simulink subsystem "SubSystemVereinzelung"  (R2020b)
settings: Solver=VariableStepAuto  StartTime=0.0  StopTime=10.0  RelTol=1e-3
libraries: simulink x6, eeGeneralControl x5
settings Model: Creator=kaebi  LastModifiedBy=kaebi

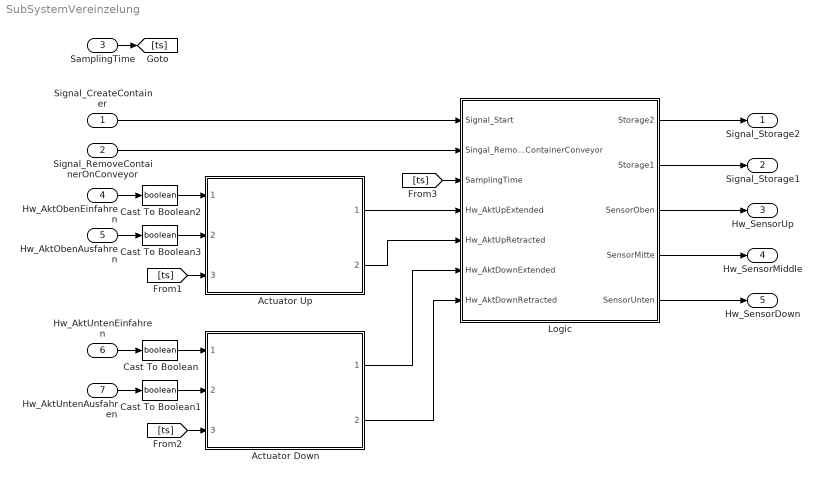
== system SubSystemVereinzelung ==
  Signal_CreateContainer : Inport
  Signal_RemoveContainerOnConveyor : Inport  Port=2
  SamplingTime : Inport  Port=3
  Hw_AktObenEinfahren : Inport  Port=4
  Hw_AktObenAusfahren : Inport  Port=5
  Hw_AktUntenEinfahren : Inport  Port=6
  Hw_AktUntenAusfahren : Inport  Port=7
  Actuator Down : Subsystem  ReferencedSubsystem=SubSystemHubmagnetVereinzelung
  Actuator Up : Subsystem  ReferencedSubsystem=SubSystemHubmagnetVereinzelung
  Cast To Boolean{,1..3} (4 alike) : DataTypeConversion  OutDataTypeStr=boolean
  Logic : Subsystem
  Signal_Storage2 : Outport
  Signal_Storage1 : Outport  Port=2
  Hw_SensorUp : Outport  Port=3
  Hw_SensorMiddle : Outport  Port=4
  Hw_SensorDown : Outport  Port=5
  wires:
  [ts] -> Actuator Up/3
  [ts] -> Actuator Down/3
  SamplingTime/1 -> [ts]
  Logic/5(SensorUnten) -> Hw_SensorDown/1
  Logic/4(SensorMitte) -> Hw_SensorMiddle/1
  Logic/3(SensorOben) -> Hw_SensorUp/1
  Logic/2(Storage1) -> Signal_Storage1/1
  Logic/1(Storage2) -> Signal_Storage2/1
  Signal_CreateContainer/1 -> Logic/1(Signal_Start)
  [ts] -> Logic/3(SamplingTime)
  Signal_RemoveContainerOnConveyor/1 -> Logic/2(Singal_RemoveContainerConveyor)
  Actuator Up/1 -> Logic/4(Hw_AktUpExtended)
  Actuator Up/2 -> Logic/5(Hw_AktUpRetracted)
  Actuator Down/1 -> Logic/6(Hw_AktDownExtended)
  Actuator Down/2 -> Logic/7(Hw_AktDownRetracted)
  Hw_AktObenEinfahren/1 -> Cast To Boolean2/1
  Hw_AktObenAusfahren/1 -> Cast To Boolean3/1
  Cast To Boolean2/1 -> Actuator Up/1
  Cast To Boolean3/1 -> Actuator Up/2
  Hw_AktUntenEinfahren/1 -> Cast To Boolean/1
  Hw_AktUntenAusfahren/1 -> Cast To Boolean1/1
  Cast To Boolean1/1 -> Actuator Down/2
  Cast To Boolean/1 -> Actuator Down/1

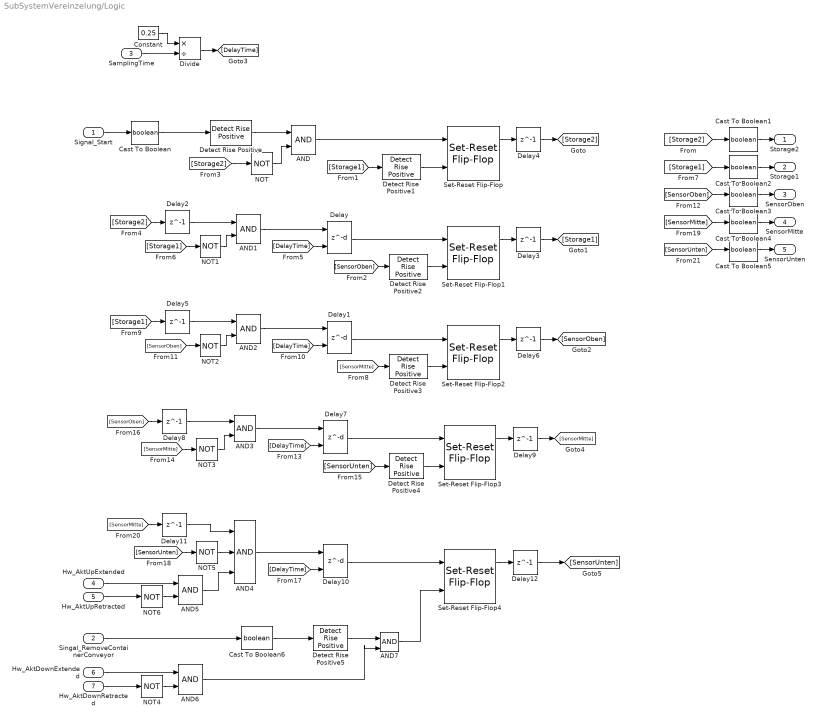
== system SubSystemVereinzelung/Logic ==
  Signal_Start : Inport
  Singal_RemoveContainerConveyor : Inport  Port=2
  SamplingTime : Inport  Port=3
  Hw_AktUpExtended : Inport  Port=4
  Hw_AktUpRetracted : Inport  Port=5
  Hw_AktDownExtended : Inport  Port=6
  Hw_AktDownRetracted : Inport  Port=7
  AND{,1..3,5..7} (7 alike) : Logic  IconShape=distinctive  AllPortsSameDT=off  OutDataTypeStr=boolean
  AND4 : Logic  Inputs=3  IconShape=distinctive  AllPortsSameDT=off  OutDataTypeStr=boolean
  Cast To Boolean{,1..6} (7 alike) : DataTypeConversion  OutDataTypeStr=boolean
  Constant : Constant  Value=0.25
  Delay{,1,7,10} (4 alike) : Delay  DelayLengthSource=Input port  DelayLengthUpperLimit=2500
      settings: InputPortMap=u0,p1
  Delay{2..6,8..9,11..12} (9 alike) : Delay  DelayLength=1
  Detect Rise Positive{,1..5} (6 alike) : simulink/Logic and Bit Operations/Detect Rise Positive  vinit=0  OutDataTypeStr=boolean
  Divide : Product  Inputs=*/
  NOT{,1..6} (7 alike) : Logic  Operator=NOT  IconShape=distinctive  AllPortsSameDT=off  OutDataTypeStr=boolean
  Set-Reset Flip-Flop{,1..4} (5 alike) : eeGeneralControl/Set-Reset Flip-Flop  LabelModeActiveChoice=Discrete  UndefState=Set  Q0=0  Ts=-1
      settings: SourceProductBaseCode=PS
  Storage2 : Outport
  Storage1 : Outport  Port=2
  SensorOben : Outport  Port=3
  SensorMitte : Outport  Port=4
  SensorUnten : Outport  Port=5
  wires:
  Hw_AktDownExtended/1 -> AND6/1
  Hw_AktDownRetracted/1 -> NOT4/1
  NOT4/1 -> AND6/2
  Hw_AktUpExtended/1 -> AND5/1
  Hw_AktUpRetracted/1 -> NOT6/1
  NOT6/1 -> AND5/2
  AND6/1 -> AND7/2
  AND5/1 -> AND4/3
  Detect Rise Positive5/1 -> AND7/1
  AND7/1 -> Set-Reset Flip-Flop4/2
  Cast To Boolean/1 -> Detect Rise Positive/1
  [SensorMitte] -> Detect Rise Positive3/1
  Detect Rise Positive3/1 -> Set-Reset Flip-Flop2/2
  Detect Rise Positive2/1 -> Set-Reset Flip-Flop1/2
  [SensorOben] -> Detect Rise Positive2/1
  Detect Rise Positive1/1 -> Set-Reset Flip-Flop/2
  [Storage1] -> Detect Rise Positive1/1
  Detect Rise Positive4/1 -> Set-Reset Flip-Flop3/2
  [SensorUnten] -> Detect Rise Positive4/1
  [SensorMitte] -> Delay11/1
  [DelayTime] -> Delay10/2
  Delay11/1 -> AND4/1
  AND4/1 -> Delay10/1
  NOT5/1 -> AND4/2
  [SensorUnten] -> NOT5/1
  Delay10/1 -> Set-Reset Flip-Flop4/1
  Delay12/1 -> [SensorUnten]
  Set-Reset Flip-Flop4/1 -> Delay12/1
  Set-Reset Flip-Flop3/1 -> Delay9/1
  Delay9/1 -> [SensorMitte]
  Delay7/1 -> Set-Reset Flip-Flop3/1
  [SensorMitte] -> NOT3/1
  NOT3/1 -> AND3/2
  AND3/1 -> Delay7/1
  Delay8/1 -> AND3/1
  [DelayTime] -> Delay7/2
  [SensorOben] -> Delay8/1
  [Storage1] -> Delay5/1
  [DelayTime] -> Delay1/2
  Delay5/1 -> AND2/1
  AND2/1 -> Delay1/1
  NOT2/1 -> AND2/2
  [SensorOben] -> NOT2/1
  Delay1/1 -> Set-Reset Flip-Flop2/1
  Delay6/1 -> [SensorOben]
  Set-Reset Flip-Flop2/1 -> Delay6/1
  Set-Reset Flip-Flop1/1 -> Delay3/1
  Delay3/1 -> [Storage1]
  Delay4/1 -> [Storage2]
  Delay/1 -> Set-Reset Flip-Flop1/1
  [Storage1] -> NOT1/1
  NOT1/1 -> AND1/2
  AND1/1 -> Delay/1
  Delay2/1 -> AND1/1
  [DelayTime] -> Delay/2
  [Storage2] -> Delay2/1
  Divide/1 -> [DelayTime]
  [Storage2] -> NOT/1
  AND/1 -> Set-Reset Flip-Flop/1
  Set-Reset Flip-Flop/1 -> Delay4/1
  SamplingTime/1 -> Divide/2
  Constant/1 -> Divide/1
  NOT/1 -> AND/2
  Detect Rise Positive/1 -> AND/1
  Signal_Start/1 -> Cast To Boolean/1
  [Storage2] -> Cast To Boolean1/1
  Cast To Boolean1/1 -> Storage2/1
  [SensorUnten] -> Cast To Boolean5/1
  [SensorMitte] -> Cast To Boolean4/1
  [SensorOben] -> Cast To Boolean3/1
  [Storage1] -> Cast To Boolean2/1
  Cast To Boolean2/1 -> Storage1/1
  Cast To Boolean3/1 -> SensorOben/1
  Cast To Boolean4/1 -> SensorMitte/1
  Cast To Boolean5/1 -> SensorUnten/1
  Cast To Boolean6/1 -> Detect Rise Positive5/1
  Singal_RemoveContainerConveyor/1 -> Cast To Boolean6/1
